simulink model "QPSK"  (R2021a)
settings: Solver=VariableStepAuto  StartTime=0.0  StopTime=10.0  RelTol=1e-3
libraries: commdigbbndpm3 x2, commchan3 x1, commsink2 x1, commrandsrc3 x1
settings Model: Creator=Bharat Gunhalkar  LastModifiedBy=Bharat Gunhalkar

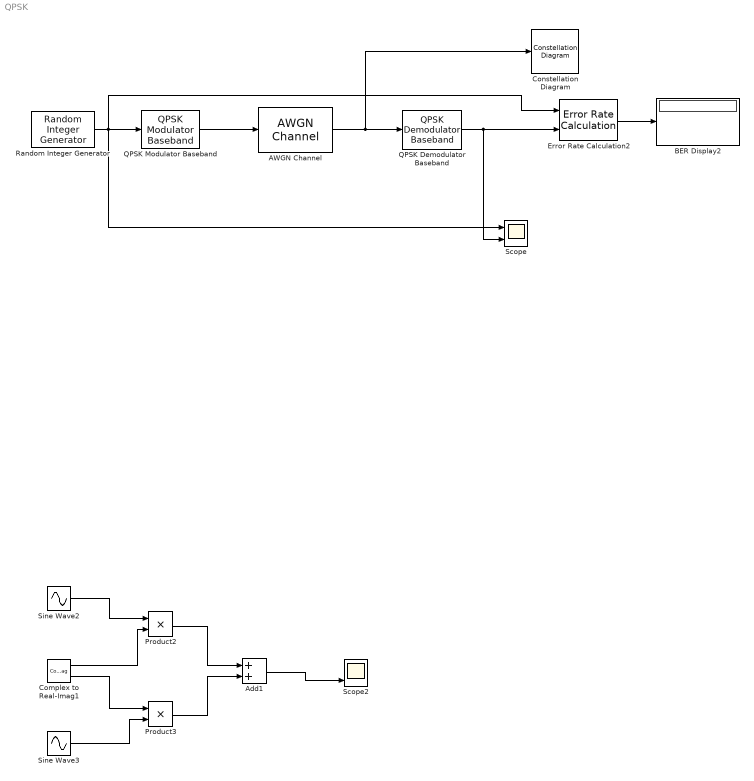
== system QPSK ==
  AWGN Channel : commchan3/AWGN Channel  InputProcessing=Columns as channels (frame based)  seed=67  noiseMode="Signal to noise ratio  (Eb/No)"  EbNodB=1  EsNodB=10  SNRdB=10  bitsPerSym=2  Ps=1  Tsym=1  variance=1
  Add1 : Sum
  BER Display2 : Display
  Complex to Real-Imag1 : ComplexToRealImag
  Constellation Diagram : ConstellationDiagram
  Error Rate Calculation2 : commsink2/Error Rate Calculation  N=0  st_delay=0  cp_mode=Entire frame  subframe=[]  PMode=Port  WsName=ErrorVec  RsMode2=off  stop=off  numErr=100  maxBits=1e6
  Product2 : Product
  Product3 : Product
  QPSK Demodulator Baseband : commdigbbndpm3/QPSK Demodulator Baseband  OutType=Integer  DecType=Hard decision  VarSource=Dialog  Variance=1  Dec=Gray  Ph=pi/4  outDtype1=Inherit via internal rule  outDtype2=Inherit via internal rule  derotateFactorWordLen=16  derotateFactorDataTypeStr=Inherit: Same word length as input  derotateFactorLastDataTypeStr=Inherit: Same word length as input
  QPSK Modulator Baseband : commdigbbndpm3/QPSK Modulator Baseband  InType=Integer  Enc=Gray  Ph=pi/4  outDtype=double  outWordLen=16  outUDDataType=sfix(16)  outFracLenMode=Best precision  outFracLen=15  outDataTypeStr=double  outLastDataTypeStr=double
  Random Integer Generator : commrandsrc3/Random Integer Generator  SetSize=4  SeedSource=Auto  Seed=0  SampleTime=1  SamplesPerFrame=1  OutputDataType=double  SimulateUsing=Interpreted execution
  Scope : Scope  NumInputPorts=2
  Scope2 : Scope  NumInputPorts=3
  Sine Wave2 : Sin  Frequency=8*pi  SampleTime=0.001
  Sine Wave3 : Sin  Frequency=8*pi  Phase=pi/2  SampleTime=0.001
  wires:
  QPSK Modulator Baseband/1 -> AWGN Channel/1
  Random Integer Generator/1 -> Scope/1, Error Rate Calculation2/1, QPSK Modulator Baseband/1
  AWGN Channel/1 -> Constellation Diagram/1, QPSK Demodulator Baseband/1
  QPSK Demodulator Baseband/1 -> Error Rate Calculation2/2, Scope/2
  ? -> Scope2/1
  Add1/1 -> Scope2/3
  Sine Wave2/1 -> Product2/1
  Complex to Real-Imag1/2 -> Product3/1
  ? -> Complex to Real-Imag1/1
  Product3/1 -> Add1/2
  Complex to Real-Imag1/1 -> Product2/2
  Product2/1 -> Add1/1
  Sine Wave3/1 -> Product3/2
  ? -> Scope2/2
  Error Rate Calculation2/1 -> BER Display2/1
